simulink model "Riego_y_Fertirriego"  (R2020a)
settings: Solver=ode5  StartTime=0.0  StopTime=Inf  FixedStep=0.1  RelTol=1e-3  EnableMultiTasking=on
libraries: sldrtlib x2
Description:
  | Water Tank Model with Dashboard
  | 
  | The example model "sldrtex_dashboard" shows a real-time model of a water tank
  | controlled by dashboard controls.  You can change the inputs to the plant using
  | the knobs and observe the response on the gauges.
  | 
  | How to run this model in Normal Mode:
  | 
  | 1) Double-click the orange button to switch to Normal Mode if needed.
  | 2) Start the real-time execution using Simulation->Run.
  | 3) Change the input flow and output valve values by the dashboard controls and observe
  |    the results on the dashboard gauges.
  | 
  | How to run this model in External Mode:
  | 
  | 1) Double-click the orange button to switch to External Mode if needed.
  | 2) Start the real-time execution using Simulation->Run. The model will automatically
  |    build, connect to Simulink in External Mode and start.
  | 3) Change the input flow and output valve values by the dashboard controls and observe
  |    the results on the dashboard gauges.
settings Model: ExtModeTrigDuration=101  Creator=The MathWorks, Inc.  LastModifiedBy=Maria Vera Tudela
settings SolverCC: AutoInsertRateTranBlk=on
settings DataIOCC: LimitDataPoints=on  SaveFormat=Array  ReturnWorkspaceOutputs=off  SignalLoggingName=logsOut
settings OptimizationCC: ExpressionDepthLimit=2147483647  InitFltsAndDblsToZero=on  EfficientMapNaN2IntZero=off  LifeSpan=inf
settings DebuggingCC: UnderspecifiedInitializationDetection=Classic  MergeDetectMultiDrivingBlocksExec=none  SignalResolutionControl=TryResolveAllWithWarning  FcnCallInpInsideContextMsg=warning  AllowSymbolicDim=off  StateNameClashWarn=warning  SymbolicDimsDataTypeCodeGenerationDiagnostic=none  SFUnexpectedBacktrackingDiag=warning  SFNoUnconditionalDefaultTransitionDiag=warning  SFExecutionAtInitializationDiag=none  ArithmeticOperatorsInVariantConditions=warning
settings HardwareCC: TargetBitPerLong=64  TargetBitPerPointer=64  TargetBitPerSizeT=64  TargetBitPerPtrDiffT=64  TargetIntDivRoundTo=Zero  TargetEndianess=LittleEndian  TargetWordSize=64  TargetHWDeviceType=Intel->x86-64
settings ModelReferenceCC: PropagateSignalLabelsOutOfModel=off
settings SFSimCC: SimUseLocalCustomCode=off
settings RTWCC: Description=Simulink Desktop Real-Time  SystemTargetFile=sldrt.tlc  TemplateMakefile=sldrt.tmf  RTWUseLocalCustomCode=off  RTWCompilerOptimization=on
settings CodeAppCC: MaxIdLength=95  StateflowObjectComments=on
settings SimulinkDesktopRealTimeCC: TargetPreCompLibLocation=C:\Program Files\MATLAB\R2020a\toolbox\sldrt\lib\win64  TargetLangStandard=C89/C90 (ANSI)  SupportVariableSizeSignals=off
settings ConfigComp: CovMetricSettings=dw  CovHtmlReporting=on  CovSaveCumulativeToWorkspaceVar=on  CovSaveSingleToWorkspaceVar=on  CovShowResultsExplorer=off  CovExternalEMLEnable=off  CovSFcnEnable=off

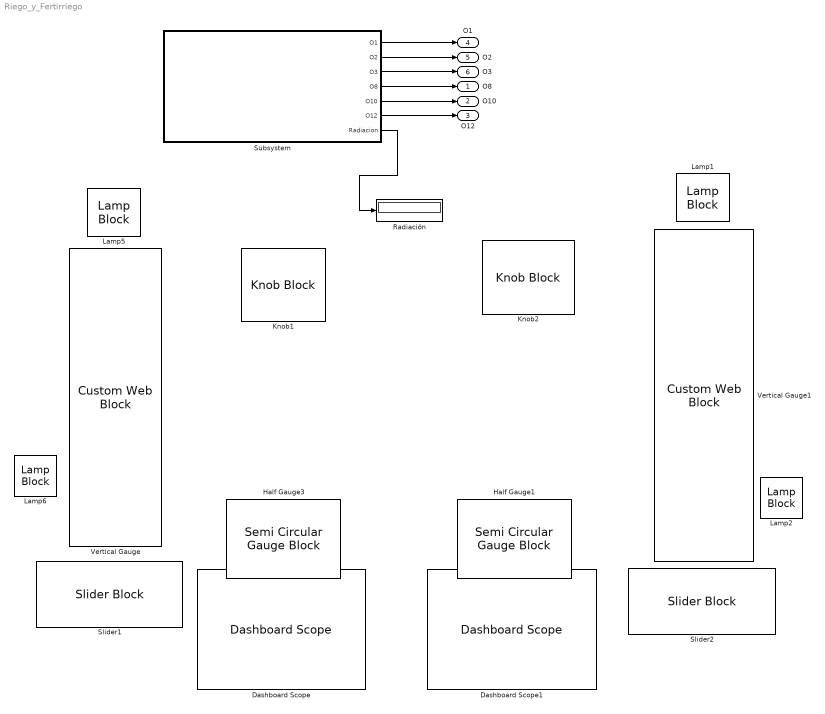
== system Riego_y_Fertirriego ==
  Dashboard Scope : DashboardScope
  Dashboard Scope1 : DashboardScope
  Half Gauge1 : SemiCircularGaugeBlock
  Half Gauge3 : SemiCircularGaugeBlock  ScaleMax=14
  Knob1 : KnobBlock  ScaleMax=14
  Knob2 : KnobBlock
  Lamp{1..2,5..6} (4 alike) : LampBlock
  Radiación : Display
  Slider1 : SliderBlock  ScaleMax=30
  Slider2 : SliderBlock  ScaleMax=30
  Subsystem : Subsystem
  Vertical Gauge : CustomWebBlock  ShowInitialText=on  Configuration="{\"components\":[{\"name\":\"LinearScaleComponent\",\"settings\":{\"bounds\":{\"max\":40,\"min\":0,\"tickInterval\":\"auto\"},\"labelColor\":[250,245,199],\"labelFont\":{\"font\":\"Arial\",\"fontSize\":12},\"labelTransparency\":1,\"needleImage\":{\"size\":[21,75],\"src\":\"data:image\\/svg+xml;base64,PHN2ZyB4bWxucz0iaHR0cDovL3d3dy53My5vcmcvMjAwMC9zdmciIHhtbG5zOnhsaW5rPSJodHRwOi8vd3d3LnczLm9yZy8xOTk5L3hsaW5rIiB2aWV3Qm94PSIwIDAgMjEgNzUiPjxkZWZzPjxzdHlsZT4uY2xzLTF7ZmlsbDpub25lO30uY2xzLTJ7aXNvbGF0aW9uOmlzb2xhdGU7fS5jbHMtM3tjbGlwLXBhdGg6dXJsKCNjbGlwLXBhdGgpO30uY2xzLTR7b3BhY2l0eTowLjM7bWl4LWJsZW5kLW1vZGU6bXVsdGlwbHk7fS5jbHMtNXtmaWxsOiNlYjI2Mjk7fTwvc3R5bGU+PGNsaXBQYXRoIGlkPSJjbGlwLXBhdGgiIHRyYW5zZm9y ...(+1928 chars)\",\"srcOrientation\":\"horizontal\"},\"needleOffset\":[-0.01094391244870041,0],\"needleSize\":{\"height\":0.11960078534031414,\"width\":0.7589285714285714},\"position\":[0.015887605042016806,0.06986607142857143,0.8,0.9641544117647058],\"scaleColorSize\":0.24,\"scaleColors\":[],\"scaleColorsSize\":0.2,\"tickColor\":[250,245,200],\"tickTransparency\":1,\"valueBarColor\":[23,89,176],\"valueBarSize\":0.23,\"valueBarTransparency\":1}},{\"name\":\"BackgroundImageComponent\",\"settings\":{\"image\":{\"size\":[380,101],\"src\":\"data:image\\/svg+xml;base64,PHN2ZyB4bWxucz0iaHR0cDovL3d3dy53My5vcmcvMjAwMC9zdmciIHhtbG5zOnhsaW5rPSJodHRwOi8vd3d3LnczLm9yZy8xOTk5L3hsaW5rIiB2aWV3Qm94PSIwIDAgMzgwIDEwMSI+PGRlZnM+PHN0eWxlPi5jbHMtMXtmaWxsOnVybCgjbGluZWFyLWdyYWRpZW50KTt9LmNscy0ye2ZpbGw6dXJsKCNsaW5lYXItZ3JhZGllbnQtMik7fS5jbHMtM3tmaWxsOnVybCgjbGluZWFyLWdyYWRpZW50LTMpO308L3N0eWxlPjxsaW5lYXJHcmFkaWVudCBpZD0ibGluZWFyLWdyYWRpZW50IiB5MT0iNTAuNSIgeDI9IjM5OS4yOCIgeTI9IjUw ...(+2216 chars)\",\"srcOrientation\":\"horizontal\"},\"position\":[0,0,1,1],\"scaleMode\":\"0\"}}],\"settings\":{\"BindingType\":\"signal\",\"fixedAspectRatio\":\"on\",\"orientation\":\"vertical\"},\"type\":\"LinearGauge\"}"
  Vertical Gauge1 : CustomWebBlock  ShowInitialText=on  Configuration="{\"components\":[{\"name\":\"LinearScaleComponent\",\"settings\":{\"bounds\":{\"max\":40,\"min\":0,\"tickInterval\":\"auto\"},\"labelColor\":[250,245,199],\"labelFont\":{\"font\":\"Arial\",\"fontSize\":12},\"labelTransparency\":1,\"needleImage\":{\"size\":[21,75],\"src\":\"data:image\\/svg+xml;base64,PHN2ZyB4bWxucz0iaHR0cDovL3d3dy53My5vcmcvMjAwMC9zdmciIHhtbG5zOnhsaW5rPSJodHRwOi8vd3d3LnczLm9yZy8xOTk5L3hsaW5rIiB2aWV3Qm94PSIwIDAgMjEgNzUiPjxkZWZzPjxzdHlsZT4uY2xzLTF7ZmlsbDpub25lO30uY2xzLTJ7aXNvbGF0aW9uOmlzb2xhdGU7fS5jbHMtM3tjbGlwLXBhdGg6dXJsKCNjbGlwLXBhdGgpO30uY2xzLTR7b3BhY2l0eTowLjM7bWl4LWJsZW5kLW1vZGU6bXVsdGlwbHk7fS5jbHMtNXtmaWxsOiNlYjI2Mjk7fTwvc3R5bGU+PGNsaXBQYXRoIGlkPSJjbGlwLXBhdGgiIHRyYW5zZm9y ...(+1928 chars)\",\"srcOrientation\":\"horizontal\"},\"needleOffset\":[-0.01094391244870041,0],\"needleSize\":{\"height\":0.11960078534031414,\"width\":0.7589285714285714},\"position\":[0.015887605042016806,0.06986607142857143,0.8,0.9641544117647058],\"scaleColorSize\":0.24,\"scaleColors\":[],\"scaleColorsSize\":0.2,\"tickColor\":[250,245,200],\"tickTransparency\":1,\"valueBarColor\":[23,89,176],\"valueBarSize\":0.23,\"valueBarTransparency\":1}},{\"name\":\"BackgroundImageComponent\",\"settings\":{\"image\":{\"size\":[380,101],\"src\":\"data:image\\/svg+xml;base64,PHN2ZyB4bWxucz0iaHR0cDovL3d3dy53My5vcmcvMjAwMC9zdmciIHhtbG5zOnhsaW5rPSJodHRwOi8vd3d3LnczLm9yZy8xOTk5L3hsaW5rIiB2aWV3Qm94PSIwIDAgMzgwIDEwMSI+PGRlZnM+PHN0eWxlPi5jbHMtMXtmaWxsOnVybCgjbGluZWFyLWdyYWRpZW50KTt9LmNscy0ye2ZpbGw6dXJsKCNsaW5lYXItZ3JhZGllbnQtMik7fS5jbHMtM3tmaWxsOnVybCgjbGluZWFyLWdyYWRpZW50LTMpO308L3N0eWxlPjxsaW5lYXJHcmFkaWVudCBpZD0ibGluZWFyLWdyYWRpZW50IiB5MT0iNTAuNSIgeDI9IjM5OS4yOCIgeTI9IjUw ...(+2216 chars)\",\"srcOrientation\":\"horizontal\"},\"position\":[0,0,1,1],\"scaleMode\":\"0\"}}],\"settings\":{\"BindingType\":\"signal\",\"fixedAspectRatio\":\"on\",\"orientation\":\"vertical\"},\"type\":\"LinearGauge\"}"
  O8 : Outport
  O10 : Outport  Port=2
  O12 : Outport  Port=3
  O1 : Outport  Port=4
  O2 : Outport  Port=5
  O3 : Outport  Port=6
  wires:
  Subsystem/1(O1) -> O1/1
  Subsystem/2(O2) -> O2/1
  Subsystem/3(O3) -> O3/1
  Subsystem/4(O8) -> O8/1
  Subsystem/5(O10) -> O10/1
  Subsystem/6(O12) -> O12/1
  Subsystem/7(Radiacion) -> Radiación/1

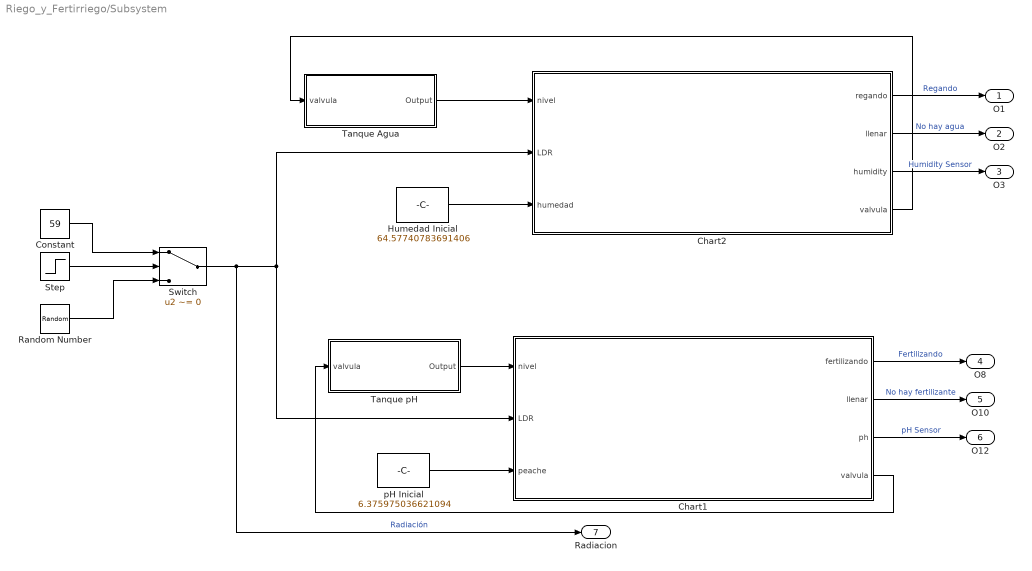
== system Riego_y_Fertirriego/Subsystem ==
  Chart1 : Stateflow chart  TreatAsAtomicUnit=on
  Chart2 : Stateflow chart  TreatAsAtomicUnit=on
  Constant : Constant  Value=59
  Humedad Inicial : Constant  Value=64.57740783691406
  Random Number : RandomNumber  Mean=59  Variance=2  SampleTime=15
  Step : Step  Time=15  Before=1  After=0  SampleTime=0
  Switch : Switch  Criteria=u2 ~= 0
  Tanque Agua : Subsystem
  Tanque pH : Subsystem
  pH Inicial : Constant  Value=6.375975036621094
  O1 : Outport
  O2 : Outport  Port=2
  O3 : Outport  Port=3
  O8 : Outport  Port=4
  O10 : Outport  Port=5
  O12 : Outport  Port=6
  Radiacion : Outport  Port=7
  wires:
  Humedad Inicial/1 -> Chart2/3(humedad)
  pH Inicial/1 -> Chart1/3(peache)
  Chart1/3(ph) -> O12/1  "pH Sensor"
  Tanque pH/1(Output) -> Chart1/1(nivel)
  Chart1/4(valvula) -> Tanque pH/1(valvula)
  Chart1/1(fertilizando) -> O8/1  "Fertilizando"
  Chart1/2(llenar) -> O10/1  "No hay fertilizante"
  Tanque Agua/1(Output) -> Chart2/1(nivel)
  Chart2/4(valvula) -> Tanque Agua/1(valvula)
  Chart2/3(humidity) -> O3/1  "Humidity Sensor"
  Chart2/2(llenar) -> O2/1  "No hay agua"
  Chart2/1(regando) -> O1/1  "Regando"
  Step/1 -> Switch/2
  Switch/1 -> Radiacion/1, Chart1/2(LDR), Chart2/2(LDR)  "Radiación"
  Random Number/1 -> Switch/3
  Constant/1 -> Switch/1

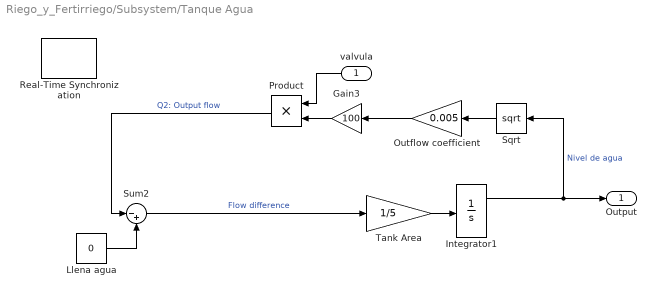
== system Riego_y_Fertirriego/Subsystem/Tanque Agua ==
  valvula : Inport
  Gain3 : Gain  Gain=100
  Integrator1 : Integrator  LimitOutput=on  UpperSaturationLimit=35  LowerSaturationLimit=0  ShowSaturationPort=on
  Llena agua : Constant  Value=0
  Outflow coefficient : Gain  Gain=0.005  SaturateOnIntegerOverflow=on  OutDataTypeStr=Inherit: Same as input  ParamDataTypeStr=Inherit: Same as input
  Product : Product
  Real-Time Synchronization : sldrtlib/Real-Time Synchronization  SampleTime=0.1  MaxMissedTicks=Inf  ShowMissedTicks=off  YieldWhenWaiting=off
  Sqrt : Sqrt  SaturateOnIntegerOverflow=on
  Sum2 : Sum  Inputs=|-+
  Tank Area : Gain  Gain=1/5  SaturateOnIntegerOverflow=on  OutDataTypeStr=Inherit: Same as input  ParamDataTypeStr=Inherit: Same as input
  Output : Outport
  wires:
  Sum2/1 -> Tank Area/1  "Flow difference"
  Integrator1/1 -> Output/1, Sqrt/1  "Nivel de agua"
  Product/1 -> Sum2/1  "Q2: Output flow"
  Sqrt/1 -> Outflow coefficient/1
  Llena agua/1 -> Sum2/2
  Tank Area/1 -> Integrator1/1
  Outflow coefficient/1 -> Gain3/1
  Gain3/1 -> Product/2
  valvula/1 -> Product/1

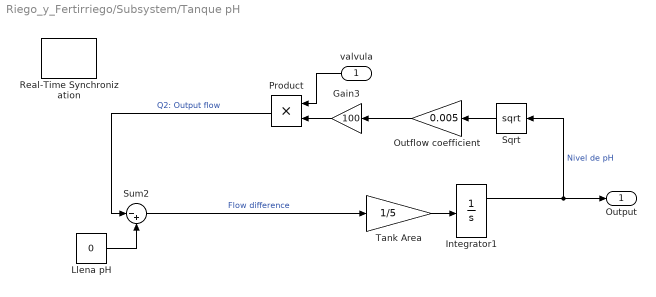
== system Riego_y_Fertirriego/Subsystem/Tanque pH ==
  valvula : Inport
  Gain3 : Gain  Gain=100
  Integrator1 : Integrator  LimitOutput=on  UpperSaturationLimit=35  LowerSaturationLimit=0  ShowSaturationPort=on
  Llena pH : Constant  Value=0
  Outflow coefficient : Gain  Gain=0.005  SaturateOnIntegerOverflow=on  OutDataTypeStr=Inherit: Same as input  ParamDataTypeStr=Inherit: Same as input
  Product : Product
  Real-Time Synchronization : sldrtlib/Real-Time Synchronization  SampleTime=0.1  MaxMissedTicks=Inf  ShowMissedTicks=off  YieldWhenWaiting=off
  Sqrt : Sqrt  SaturateOnIntegerOverflow=on
  Sum2 : Sum  Inputs=|-+
  Tank Area : Gain  Gain=1/5  SaturateOnIntegerOverflow=on  OutDataTypeStr=Inherit: Same as input  ParamDataTypeStr=Inherit: Same as input
  Output : Outport
  wires:
  Sum2/1 -> Tank Area/1  "Flow difference"
  Integrator1/1 -> Output/1, Sqrt/1  "Nivel de pH"
  Product/1 -> Sum2/1  "Q2: Output flow"
  Sqrt/1 -> Outflow coefficient/1
  Llena pH/1 -> Sum2/2
  Tank Area/1 -> Integrator1/1
  Outflow coefficient/1 -> Gain3/1
  Gain3/1 -> Product/2
  valvula/1 -> Product/1

== stateflow chart Riego_y_Fertirriego/Subsystem/Chart1 ==
  state INICIO
    entry:
    cod=0;
    ph=peache;
    fertilizando=0;
    llenar=0;
    during:
    ph=ph-0.05
    valvula=0
    exit:
    cod=1;
  state FERTILIZAR
    entry:
    cod=1;
    fertilizando=1;
    llenar=0;
    during:
    ph=ph+0.1
    valvula=1
    exit:
    cod=2;
  state PH
    entry:
    fertilizando=0;
    llenar=1;
    during:
    ph=0
    valvula=0
  state PH_BAJA_LDR
    entry:
    cod=0;
    fertilizando=0;
    llenar=0;
    during:
    ph=ph-0.05
    valvula=0
    exit:
    cod=1;
  state TANQUE_VACIO
    entry:
    fertilizando=0;
    llenar=1;
    during:
    ph=ph-0.05
    valvula=0
  state PH_9_BAJA
    entry:
    cod=2;
    fertilizando=0;
    llenar=0;
    during:
    ph=ph-0.05
    valvula=0
    exit:
    cod=1;
  state LLENAR_TANQUE
    entry:
    fertilizando=0;
    llenar=1;
    during:
    ph=ph-0.05
    valvula=0
    exit:
    cod=1;
  state PH1
    ph=0
    valvula=0
  state APAGAR
    entry:
    fertilizando=0;
    llenar=0;
    during:
    valvula=0
    ph=ph-0.05
  (default) -> INICIO [order 2] : [LDR<=60]
  (junction 3) -> FERTILIZAR : [nivel>=5]
  INICIO -> PH_9_BAJA [order 3] : [ph>=7]
  PH -> FERTILIZAR : [nivel>=5]
  INICIO -> (junction 3) [order 2] : [ph<7]
  PH_BAJA_LDR -> (junction 3) [order 3] : [ph<7]
  TANQUE_VACIO -> PH [order 1] : [ph<=0]
  INICIO -> TANQUE_VACIO [order 1] : [nivel<5]
  (junction 53) -> FERTILIZAR : [ph<7]
  LLENAR_TANQUE -> PH [order 2] : [ph<=0]
  FERTILIZAR -> APAGAR [order 2] : [LDR>60]
  TANQUE_VACIO -> (junction 53) [order 2] : [nivel>=15]
  FERTILIZAR -> LLENAR_TANQUE [order 3] : [nivel<5]
  PH_9_BAJA -> FERTILIZAR [order 3] : [ph<7]/{cod=1}
  FERTILIZAR -> PH_9_BAJA [order 1] : [ph>=9]/{cod=2}
  PH_BAJA_LDR -> TANQUE_VACIO [order 1] : [nivel<5]
  PH_BAJA_LDR -> PH_9_BAJA [order 2] : [ph>=7]
  APAGAR -> PH_BAJA_LDR [order 1] : [LDR<=60]
  PH1 -> PH_BAJA_LDR : [LDR<=60]
  (default) -> APAGAR [order 1] : [LDR>60]
  APAGAR -> PH1 [order 2] : [ph<=0]
  LLENAR_TANQUE -> PH_9_BAJA [order 1] : [nivel>15]
  PH_9_BAJA -> LLENAR_TANQUE [order 1] : [nivel<5]
  PH_9_BAJA -> APAGAR [order 2] : [LDR>60]
  data: nivel input; cod local; fertilizando output; llenar output; LDR input; peache input; ph output; valvula output

== stateflow chart Riego_y_Fertirriego/Subsystem/Chart2 ==
  state INICIO
    entry:
    cod=0;
    humidity=humedad;
    regando=0;
    llenar=0;
    during:
    humidity=humidity-0.01
    valvula=0
    exit:
    cod=1;
  state HUMEDAD
    entry:
    regando=0;
    llenar=1;
    during:
    humidity=0
    valvula=0
  state TANQUE_VACIO
    entry:
    regando=0;
    llenar=1;
    during:
    humidity=humidity-0.01
    valvula=0
  state HUME_BAJA_LDR
    entry:
    cod=0;
    regando=0;
    llenar=0;
    during:
    humidity=humidity-0.1
    valvula=0
    exit:
    cod=1;
  state TANQUE_LLENO
    entry:
    llenar=0;
    during:
    humidity=humidity-0.01
  state REGAR
    entry:
    cod=1;
    regando=1;
    llenar=0;
    during:
    humidity=humidity+0.1
    valvula=1
    exit:
    cod=2;
  state APAGAR
    entry:
    regando=0;
    llenar=0;
    during:
    valvula=0
    humidity=humidity-0.1
  state HUMEDAD2
    humidity=0
    valvula=0
  state LLENAR_TANQUE
    entry:
    regando=0;
    llenar=1;
    during:
    humidity=humidity-0.1
    valvula=0
    exit:
    cod=1;
  state HUME_80_BAJA
    entry:
    cod=2;
    regando=0;
    llenar=0;
    during:
    humidity=humidity-0.1
    valvula=0
    exit:
    cod=1;
  (default) -> INICIO [order 2] : [LDR<=60]
  INICIO -> HUME_80_BAJA [order 3] : [humidity>=80]
  TANQUE_VACIO -> HUMEDAD [order 1] : [humidity<=0]
  INICIO -> (junction 3) [order 2] : [humidity<20]
  HUMEDAD -> REGAR [order 1] : [nivel>=5]
  LLENAR_TANQUE -> HUMEDAD [order 2] : [humidity<=0]
  HUMEDAD -> APAGAR [order 2] : [LDR>60]
  INICIO -> TANQUE_VACIO [order 1] : [nivel<5]
  HUME_BAJA_LDR -> TANQUE_VACIO [order 2] : [nivel<5]
  TANQUE_VACIO -> TANQUE_LLENO [order 2] : [nivel>=15]
  TANQUE_VACIO -> APAGAR [order 3] : [LDR>60]
  HUME_BAJA_LDR -> (junction 3) [order 1] : [humidity<20]
  (junction 3) -> REGAR : [nivel>=5]
  HUME_BAJA_LDR -> HUME_80_BAJA [order 3] : [humidity>=80]
  TANQUE_LLENO -> REGAR [order 1] : [humidity<20]
  HUMEDAD2 -> HUME_BAJA_LDR : [LDR<=60]
  APAGAR -> HUME_BAJA_LDR [order 1] : [LDR<=60]
  TANQUE_LLENO -> APAGAR [order 2] : [LDR>60]
  REGAR -> APAGAR [order 3] : [LDR>60]
  (default) -> APAGAR [order 1] : [LDR>60]
  REGAR -> LLENAR_TANQUE [order 1] : [nivel<5]
  HUME_80_BAJA -> REGAR [order 3] : [humidity<20]/{cod=1}
  REGAR -> HUME_80_BAJA [order 2] : [humidity>=80]/{cod=2}
  APAGAR -> HUMEDAD2 [order 2] : [humidity<=0]
  LLENAR_TANQUE -> HUME_80_BAJA [order 1] : [nivel>15]
  HUME_80_BAJA -> APAGAR [order 2] : [LDR>60]
  HUME_80_BAJA -> LLENAR_TANQUE [order 1] : [nivel<5]
  data: nivel input; cod local; regando output; llenar output; LDR input; humedad input; humidity output; valvula output
